simulink model "DA42_Model"  (Simulink 7.5)
settings: Solver=ode45  StartTime=0.0  StopTime=inf  RelTol=1e-3
undefined symbols (not defined in the file or in its folder): BHP_A, BHP_B, CP_norm, Pr_Alt, PropEff_norm, S
libraries: simulink_extras x4, aerolibatmos2 x2
(part 1 of 3)
settings Model: Creator=eagle  LastModifiedBy=eagle

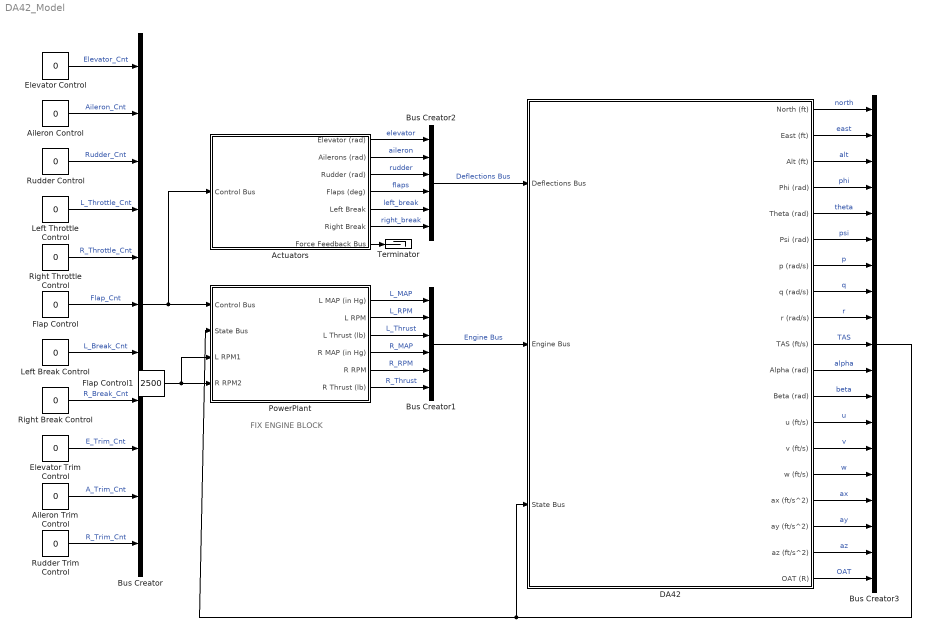
== system DA42_Model ==
  note: FIX ENGINE BLOCK
  Actuators : Subsystem
  Aileron Control : Constant  Value=0  OutDataType=sfix(16)  OutScaling=2^0
  Aileron Trim Control : Constant  Value=0  OutDataType=sfix(16)  OutScaling=2^0
  Bus Creator : BusCreator  Inputs='Elevator_Cnt','Aileron_Cnt','Rudder_Cnt','L_Throttle_Cnt','R_Throttle_Cnt','Flap_Cnt','L_Break_Cnt','R_Break_Cnt','E_Trim_Cnt','A_Trim_Cnt','R_Trim_Cnt'
  Bus Creator1 : BusCreator  Inputs='L_MAP','L_RPM','L_Thrust','R_MAP','R_RPM','R_Thrust'
  Bus Creator2 : BusCreator  Inputs='elevator','aileron','rudder','flaps','left_break','right_break'
  Bus Creator3 : BusCreator  Inputs='north','east','alt','phi','theta','psi','p','q','r','TAS','alpha','beta','u','v','w','ax','ay','az','OAT'
  DA42 : Subsystem  mask(6DoF Simulator){x0=[165               0      21.4681707               0               0               0               0     0.129383298               0               0               0           10000], Geom=[175.3 44 4.17 3935 6163.91 1029.56 5646.43 0], cg=[-7.8750 0 0.856], ac=[-7.8750 0 0.856], engR=[-3.585  5.338 0], engL=[-3.585 -5.338 0], thrustPercent=[0.966898954 0 -0.033101045], liftder=[0 0 0 -41.807 0.7530], sideder=[-0.28 -0.3940], rollder=[-0.13 -0.76 0.1180 -0.19 -0.0095], pitchder=[-0.51 0 -9.67 -0.57], yawder=[0.058 -0.11 -0.114 -0.0033 0.077]}
      mask prompts: x0 "Initial Conditions: [u v w p q r bank pitch heading N E H]"; Geom "Geometry: [S b cbar W Jx Jy Jz Jxz]"; cg "CG Location: [x y z]"; ac "AC Location: [x y z]"; engR "Right Engine Location: [x y z]"; engL "Left Engine Location: [x y z]"; thrustPercent "Thrust Percent: [x y z]"; liftder "Lift Derivatives: [CLo CLa CLadot CLq CLde]"; sideder "Side Force Derivatives: [CYb CYdr]"; rollder "Rolling Moment Derivatives: [CLb CLp CLr CLda CLdr]"; pitchder "Pitching Moment Derivatives: [Cma Cmadot Cmq Cmde]"; yawder "Yawing Moment Derivatives: [CNb CNp CNr CNda CNdr]"
      mask help:
      | 6 Degrees of Freedom simulator.
      |
      | Control Inputs = [elevator ailerons rudder throttle] rad
      mask TabNameString: Initial Conditions,Geometry,Geometry,Geometry,Engine,Engine,Engine,Derivatives,Derivatives,Derivatives,Derivatives,Derivatives
  Elevator Control : Constant  Value=0  OutDataType=sfix(16)  OutScaling=2^0
  Elevator Trim Control : Constant  Value=0  OutDataType=sfix(16)  OutScaling=2^0
  Flap Control : Constant  Value=0  OutDataType=sfix(16)  OutScaling=2^0
  Flap Control1 : Constant  Value=2500  OutDataType=sfix(16)  OutScaling=2^0
  Left Break Control : Constant  Value=0  OutDataType=sfix(16)  OutScaling=2^0
  Left Throttle Control : Constant  Value=0  OutDataType=sfix(16)  OutScaling=2^0
  PowerPlant : Subsystem  InitFcn=|
      | pitch_Angles = 15:5:40;
      | newData1 = load('-mat', 'CP_norm');
      | % Create new variables in the base workspace from those fields.
      | vars = fieldnames(newData1);
      | for i = 1:length(vars)
      |     assignin('base', vars{i}, newData1.(vars{i}));
      | end
      | clear i newData1 vars;
      | newData1 = load('-mat', 'PropEff_norm');
      | % Create new variables in the base workspace from those fields.
      | vars = fieldnames(newData1);
      | for i = 1:length(vars)
      |     assignin('base', vars{i}, newData1.(vars{i}));
      | end
      | clear i newData1 vars;
      | %% Lycoming IO-360 ENGINE PERFORMANCE
      | MAP = 12:2:28;
      | RPM = [2000; 2200; 2400; 2600; 2700];
      | %Table1:
      |     %Known: MAP and RPM.
      |     %Output: BHP-A
      |     BHP_A = [...
      |          58.0,  65.0,  68.0,  69.7,  71.5;...
      |          67.0,  75.5,  80.5,  85.0,  86.0;...
      |          79.0,  86.0,  92.5,  97.0,  99.0;...
      |          89.0,  97.0, 105.0, 110.5, 114.5;...
      |          98.0, 108.0, 116.0, 124.0, 126.0;...
      |         108.5, 118.5, 127.0, 135.5, 139.8;...
      |         118.0, 128.0, 139.0, 148.0, 152.5;...
      |         128.0, 139.0, 149.0, 160.0, 165.0;...
      |         137.5, 148.5, 161.0, 172.0, 177.5;...
      |         ];
      | %Table 2:
      |     %Known: MAP and RPM
      |     %Output: BHP-B
      |     %Comments: Equations for the lines based on linear extrapolation for
      |     %BHP-B. Has associated Excel File: "BHB_B.xlsx" to figure out the
      |     %equations for the lines
      |     for i = 1:9
      |         BHP_B(i,:) = [...
      |             ((6.818*MAP(i)) - 55.91),...
      |             ((7.167*MAP(i)) - 55.67),...
      |             ((7.857*MAP(i)) - 62.86),...
      |             ((8.333*MAP(i)) - 63.33),...
      |             ((8.5*MAP(i)) - 63),...
      |             ];
      |     end
      |     clear i;
      | %Table 3:
      |     %Known: MAP and RPM
      |     %Output: Pressure Altitude - A
      |     Pr_Alt = [...
      |         22.80, 22.70, 26.00, 25.00, 25.00;...
      |         19.20, 19.15, 19.10, 19.05, 19.00;...
      |         15.90, 15.80, 15.70, 15.60, 15.60;...
      |         12.95, 12.90, 12.80, 12.60, 12.55;...
      |         10.30, 10.25, 10.20, 10.10, 10.05;...
      |          7.85,  7.75,  7.65,  7.55,  7.50;...
      |          5.50,  5.47,  5.30,  5.25,  5.20;...
      |          3.40,  3.30,  3.25,  3.20,  3.15;...
      |          1.30,  1.25,  1.20,  1.10,  1.05;...
      |         ];
      |     Pr_Alt = Pr_Alt * 1000;
  Right Break Control : Constant  Value=0  OutDataType=sfix(16)  OutScaling=2^0
  Right Throttle Control : Constant  Value=0  OutDataType=sfix(16)  OutScaling=2^0
  Rudder Control : Constant  Value=0  OutDataType=sfix(16)  OutScaling=2^0
  Rudder Trim Control : Constant  Value=0  OutDataType=sfix(16)  OutScaling=2^0
  Terminator : Terminator
  wires:
  Aileron Control/1 -> Bus Creator/2  "Aileron_Cnt"
  Rudder Control/1 -> Bus Creator/3  "Rudder_Cnt"
  Left Throttle Control/1 -> Bus Creator/4  "L_Throttle_Cnt"
  Right Throttle Control/1 -> Bus Creator/5  "R_Throttle_Cnt"
  Flap Control/1 -> Bus Creator/6  "Flap_Cnt"
  Left Break Control/1 -> Bus Creator/7  "L_Break_Cnt"
  Right Break Control/1 -> Bus Creator/8  "R_Break_Cnt"
  Elevator Trim Control/1 -> Bus Creator/9  "E_Trim_Cnt"
  Aileron Trim Control/1 -> Bus Creator/10  "A_Trim_Cnt"
  Rudder Trim Control/1 -> Bus Creator/11  "R_Trim_Cnt"
  Elevator Control/1 -> Bus Creator/1  "Elevator_Cnt"
  PowerPlant/1(L MAP (in Hg)) -> Bus Creator1/1  "L_MAP"
  PowerPlant/2(L RPM) -> Bus Creator1/2  "L_RPM"
  PowerPlant/3(L Thrust (lb)) -> Bus Creator1/3  "L_Thrust"
  PowerPlant/4(R MAP (in Hg)) -> Bus Creator1/4  "R_MAP"
  PowerPlant/5(R RPM) -> Bus Creator1/5  "R_RPM"
  PowerPlant/6(R Thrust (lb)) -> Bus Creator1/6  "R_Thrust"
  Actuators/1(Elevator (rad)) -> Bus Creator2/1  "elevator"
  Actuators/2(Ailerons (rad)) -> Bus Creator2/2  "aileron"
  Actuators/3(Rudder (rad)) -> Bus Creator2/3  "rudder"
  Actuators/4(Flaps (deg)) -> Bus Creator2/4  "flaps"
  Actuators/5(Left Break) -> Bus Creator2/5  "left_break"
  Actuators/6(Right Break) -> Bus Creator2/6  "right_break"
  Actuators/7(Force Feedback Bus) -> Terminator/1
  Bus Creator2/1 -> DA42/1(Deflections Bus)  "Deflections Bus"
  Bus Creator1/1 -> DA42/2(Engine Bus)  "Engine Bus"
  DA42/1(North (ft)) -> Bus Creator3/1  "north"
  DA42/2(East (ft)) -> Bus Creator3/2  "east"
  DA42/3(Alt (ft)) -> Bus Creator3/3  "alt"
  DA42/4(Phi (rad)) -> Bus Creator3/4  "phi"
  DA42/5(Theta (rad)) -> Bus Creator3/5  "theta"
  DA42/6(Psi (rad)) -> Bus Creator3/6  "psi"
  DA42/7(p (rad/s)) -> Bus Creator3/7  "p"
  DA42/8(q (rad/s)) -> Bus Creator3/8  "q"
  DA42/9(r (rad/s)) -> Bus Creator3/9  "r"
  DA42/10(TAS (ft/s)) -> Bus Creator3/10  "TAS"
  DA42/11(Alpha (rad)) -> Bus Creator3/11  "alpha"
  DA42/12(Beta (rad)) -> Bus Creator3/12  "beta"
  DA42/13(u (ft/s)) -> Bus Creator3/13  "u"
  DA42/14(v (ft/s)) -> Bus Creator3/14  "v"
  DA42/15(w (ft/s)) -> Bus Creator3/15  "w"
  DA42/16(ax (ft/s^2)) -> Bus Creator3/16  "ax"
  DA42/17(ay (ft/s^2)) -> Bus Creator3/17  "ay"
  DA42/18(az (ft/s^2)) -> Bus Creator3/18  "az"
  Bus Creator3/1 -> DA42/3(State Bus), PowerPlant/2(State Bus)
  Bus Creator/1 -> PowerPlant/1(Control Bus), Actuators/1(Control Bus)
  DA42/19(OAT (R)) -> Bus Creator3/19  "OAT"
  Flap Control1/1 -> PowerPlant/4(R RPM2), PowerPlant/3(L RPM1)

== system DA42_Model/Actuators ==
  note: Orange = SR22 = Needs Updating
  Control Bus : Inport
  Aileron Control Model : Subsystem
  Aileron Trim : Subsystem
  Bus Creator1 : BusCreator  Inputs='Stick_Force','Aileron_Torque','Pedal_Force'
  Elevator Control Model : Subsystem
  Elevator Trim : Subsystem
  Flaps : Subsystem
  Left Brake : Subsystem
  Right Brake : Subsystem
  Rudder Control Model : Subsystem
  Elevator (rad) : Outport  OutDataType=fixdt(1, 16)  OutScaling=2^0
  Ailerons (rad) : Outport  Port=2  OutDataType=fixdt(1, 16)  OutScaling=2^0
  Rudder (rad) : Outport  Port=3  OutDataType=fixdt(1, 16)  OutScaling=2^0
  Flaps (deg) : Outport  Port=4  OutDataType=fixdt(1, 16)  OutScaling=2^0
  Left Break : Outport  Port=5  OutDataType=fixdt(1, 16)  OutScaling=2^0
  Right Break : Outport  Port=6  OutDataType=fixdt(1, 16)  OutScaling=2^0
  Force Feedback Bus : Outport  Port=7  OutDataType=fixdt(1, 16)  OutScaling=2^0
  wires:
  Control Bus/1 -> Elevator Control Model/1(Elevator Control), Aileron Control Model/1(Aileron Control), Right Brake/1(R_BRK_ Control), Left Brake/1(L_BRK_ Control), Flaps/1(Flap CMD), Rudder Control Model/1(Rudder Control), Aileron Trim/1(Aileron Trim CMD), Elevator Trim/1(Elevator Trim CMD)
  Flaps/1(Flap Surface) -> Rudder Control Model/4(Flap Surface), Aileron Control Model/5(Flap Surface), Elevator Control Model/5(Flap Surface), Flaps/2(Flap Surf), Flaps (deg)/1  "flaps"
  Elevator Trim/1(Elevator Trim Position) -> Elevator Trim/4(Elev Trim Position), Elevator Control Model/2(Elevator Trim Position)
  Aileron Trim/1(Aileron Trim Position) -> Aileron Trim/4(Ail Trim Position), Aileron Control Model/2(Aileron Trim Position)
  Elevator Control Model/1(Elevator Surface) -> Elevator (rad)/1  "elevator"
  Aileron Control Model/1(Aileron Torque) -> Bus Creator1/2  "Aileron_Torque"
  Rudder Control Model/1(Pedal Force) -> Bus Creator1/3  "Pedal_Force"
  Elevator Control Model/2(Stick Force) -> Bus Creator1/1  "Stick_Force"
  Bus Creator1/1 -> Force Feedback Bus/1
  Aileron Control Model/2(Aileron Surface) -> Ailerons (rad)/1  "aileron"
  Rudder Control Model/2(Rudder Surface) -> Rudder (rad)/1  "rudder"
  Right Brake/1(R_BRK_CMD) -> Right Break/1  "right_break"
  Left Brake/1(L_BRK_CMD) -> Left Break/1  "left_break"

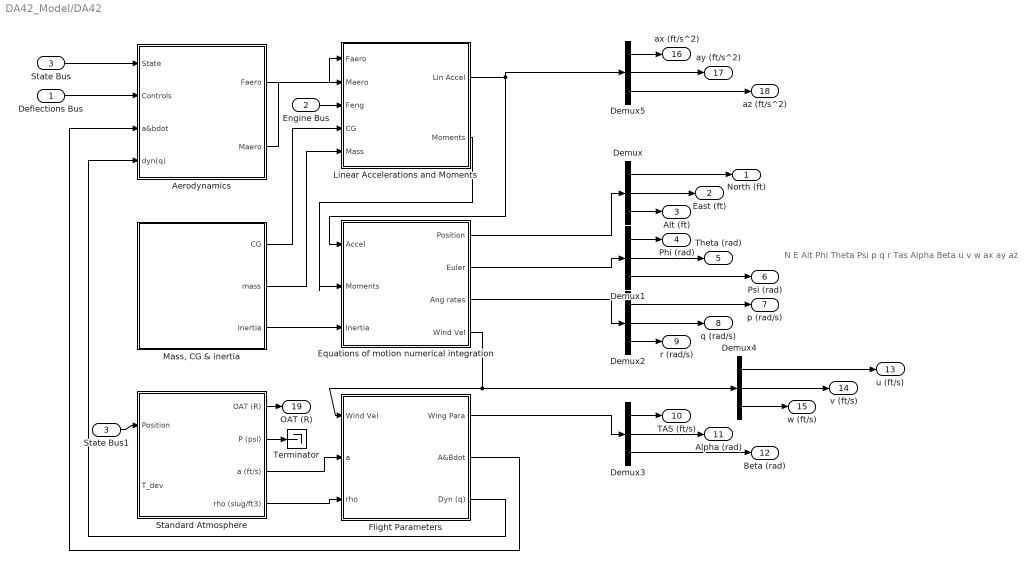
== system DA42_Model/DA42 ==
  note: N
      | E
      | Alt
      | Phi
      | Theta
      | Psi
      | p
      | q
      | r
      | Tas
      | Alpha
      | Beta
      | u
      | v
      | w
      | ax
      | ay
      | az
  Deflections Bus : Inport
  Engine Bus : Inport  Port=2
  State Bus : Inport  Port=3
  Aerodynamics : Subsystem
  Demux{,1..5} (6 alike) : Demux  Outputs=3
  "Equations of motion numerical integration " : Subsystem
  Flight Parameters : Subsystem
  Linear Accelerations and Moments : Subsystem
  "Mass, CG & inertia" : Subsystem
  Standard Atmosphere : Subsystem
  State Bus1 : InportShadow  Port=3
  Terminator : Terminator
  North (ft) : Outport
  East (ft) : Outport  Port=2
  Alt (ft) : Outport  Port=3
  Phi (rad) : Outport  Port=4
  Theta (rad) : Outport  Port=5
  Psi (rad) : Outport  Port=6
  p (rad/s) : Outport  Port=7
  q (rad/s) : Outport  Port=8
  r (rad/s) : Outport  Port=9
  TAS (ft/s) : Outport  Port=10
  Alpha (rad) : Outport  Port=11
  Beta (rad) : Outport  Port=12
  u (ft/s) : Outport  Port=13
  v (ft/s) : Outport  Port=14
  w (ft/s) : Outport  Port=15
  ax (ft/s^2) : Outport  Port=16
  ay (ft/s^2) : Outport  Port=17
  az (ft/s^2) : Outport  Port=18
  OAT (R) : Outport  Port=19
  wires:
  "Equations of motion numerical integration "/1(Position) -> Demux/1
  Flight Parameters/2(A&Bdot) -> Aerodynamics/3(a&bdot)
  Flight Parameters/3(Dyn (q)) -> Aerodynamics/4(dyn(q))
  Flight Parameters/1(Wing Para) -> Demux3/1
  "Equations of motion numerical integration "/4(Wind Vel) -> Demux4/1, Flight Parameters/1(Wind Vel)
  "Equations of motion numerical integration "/3(Ang rates) -> Demux2/1
  Linear Accelerations and Moments/1(Lin Accel) -> "Equations of motion numerical integration "/1(Accel), Demux5/1
  Deflections Bus/1 -> Aerodynamics/2(Controls)
  Aerodynamics/2(Maero) -> Linear Accelerations and Moments/2(Maero)
  Aerodynamics/1(Faero) -> Linear Accelerations and Moments/1(Faero)
  Engine Bus/1 -> Linear Accelerations and Moments/3(Feng)
  Demux/1 -> North (ft)/1
  Demux/2 -> East (ft)/1
  Demux/3 -> Alt (ft)/1
  "Equations of motion numerical integration "/2(Euler) -> Demux1/1
  Demux1/1 -> Phi (rad)/1
  Demux1/2 -> Theta (rad)/1
  Demux1/3 -> Psi (rad)/1
  Demux2/1 -> p (rad/s)/1
  Demux2/2 -> q (rad/s)/1
  Demux2/3 -> r (rad/s)/1
  Demux3/1 -> TAS (ft/s)/1
  Demux3/2 -> Alpha (rad)/1
  Demux3/3 -> Beta (rad)/1
  Demux4/1 -> u (ft/s)/1
  Demux4/2 -> v (ft/s)/1
  Demux4/3 -> w (ft/s)/1
  Demux5/1 -> ax (ft/s^2)/1
  Demux5/2 -> ay (ft/s^2)/1
  Demux5/3 -> az (ft/s^2)/1
  Linear Accelerations and Moments/2(Moments) -> "Equations of motion numerical integration "/2(Moments)
  "Mass, CG & inertia"/1(CG) -> Linear Accelerations and Moments/4(CG)
  "Mass, CG & inertia"/2(mass) -> Linear Accelerations and Moments/5(Mass)
  "Mass, CG & inertia"/3(Inertia) -> "Equations of motion numerical integration "/3(Inertia)
  Standard Atmosphere/4(rho (slug/ft3)) -> Flight Parameters/3(rho)
  Standard Atmosphere/3(a (ft/s)) -> Flight Parameters/2(a)
  State Bus/1 -> Aerodynamics/1(State)
  State Bus1/1 -> Standard Atmosphere/1(Position)
  Standard Atmosphere/1(OAT (R)) -> OAT (R)/1
  Standard Atmosphere/2(P (psi)) -> Terminator/1

== system DA42_Model/PowerPlant ==
  Control Bus : Inport
  State Bus : Inport  Port=2
  L RPM1 : Inport  Port=3
  R RPM2 : Inport  Port=4
  Bus Selector : BusSelector  OutputSignals=L_Throttle_Cnt,R_Throttle_Cnt
  Bus Selector1 : BusSelector  OutputSignals=alt,OAT,TAS
  Bus Selector2 : BusSelector  OutputSignals=alt,OAT
  Lycoming IO-1 : Subsystem  InitFcn=|
      | pitch_Angles = 15:5:40;
      | newData1 = load('-mat', 'CP_norm');
      | % Create new variables in the base workspace from those fields.
      | vars = fieldnames(newData1);
      | for i = 1:length(vars)
      |     assignin('base', vars{i}, newData1.(vars{i}));
      | end
      | clear i newData1 vars;
      | newData1 = load('-mat', 'PropEff_norm');
      | % Create new variables in the base workspace from those fields.
      | vars = fieldnames(newData1);
      | for i = 1:length(vars)
      |     assignin('base', vars{i}, newData1.(vars{i}));
      | end
      | clear i newData1 vars;
      | %% Lycoming IO-360 ENGINE PERFORMANCE
      | MAP = 12:2:28;
      | RPM = [2000; 2200; 2400; 2600; 2700];
      | %Table1:
      |     %Known: MAP and RPM.
      |     %Output: BHP-A
      |     BHP_A = [...
      |          58.0,  65.0,  68.0,  69.7,  71.5;...
      |          67.0,  75.5,  80.5,  85.0,  86.0;...
      |          79.0,  86.0,  92.5,  97.0,  99.0;...
      |          89.0,  97.0, 105.0, 110.5, 114.5;...
      |          98.0, 108.0, 116.0, 124.0, 126.0;...
      |         108.5, 118.5, 127.0, 135.5, 139.8;...
      |         118.0, 128.0, 139.0, 148.0, 152.5;...
      |         128.0, 139.0, 149.0, 160.0, 165.0;...
      |         137.5, 148.5, 161.0, 172.0, 177.5;...
      |         ];
      | %Table 2:
      |     %Known: MAP and RPM
      |     %Output: BHP-B
      |     %Comments: Equations for the lines based on linear extrapolation for
      |     %BHP-B. Has associated Excel File: "BHB_B.xlsx" to figure out the
      |     %equations for the lines
      |     for i = 1:9
      |         BHP_B(i,:) = [...
      |             ((6.818*MAP(i)) - 55.91),...
      |             ((7.167*MAP(i)) - 55.67),...
      |             ((7.857*MAP(i)) - 62.86),...
      |             ((8.333*MAP(i)) - 63.33),...
      |             ((8.5*MAP(i)) - 63),...
      |             ];
      |     end
      |     clear i;
      | %Table 3:
      |     %Known: MAP and RPM
      |     %Output: Pressure Altitude - A
      |     Pr_Alt = [...
      |         22.80, 22.70, 26.00, 25.00, 25.00;...
      |         19.20, 19.15, 19.10, 19.05, 19.00;...
      |         15.90, 15.80, 15.70, 15.60, 15.60;...
      |         12.95, 12.90, 12.80, 12.60, 12.55;...
      |         10.30, 10.25, 10.20, 10.10, 10.05;...
      |          7.85,  7.75,  7.65,  7.55,  7.50;...
      |          5.50,  5.47,  5.30,  5.25,  5.20;...
      |          3.40,  3.30,  3.25,  3.20,  3.15;...
      |          1.30,  1.25,  1.20,  1.10,  1.05;...
      |         ];
      |     Pr_Alt = Pr_Alt * 1000;
  Lycoming IO-360 : Subsystem  InitFcn=|
      | pitch_Angles = 15:5:40;
      | newData1 = load('-mat', 'CP_norm');
      | % Create new variables in the base workspace from those fields.
      | vars = fieldnames(newData1);
      | for i = 1:length(vars)
      |     assignin('base', vars{i}, newData1.(vars{i}));
      | end
      | clear i newData1 vars;
      | newData1 = load('-mat', 'PropEff_norm');
      | % Create new variables in the base workspace from those fields.
      | vars = fieldnames(newData1);
      | for i = 1:length(vars)
      |     assignin('base', vars{i}, newData1.(vars{i}));
      | end
      | clear i newData1 vars;
      | %% Lycoming IO-360 ENGINE PERFORMANCE
      | MAP = 12:2:28;
      | RPM = [2000; 2200; 2400; 2600; 2700];
      | %Table1:
      |     %Known: MAP and RPM.
      |     %Output: BHP-A
      |     BHP_A = [...
      |          58.0,  65.0,  68.0,  69.7,  71.5;...
      |          67.0,  75.5,  80.5,  85.0,  86.0;...
      |          79.0,  86.0,  92.5,  97.0,  99.0;...
      |          89.0,  97.0, 105.0, 110.5, 114.5;...
      |          98.0, 108.0, 116.0, 124.0, 126.0;...
      |         108.5, 118.5, 127.0, 135.5, 139.8;...
      |         118.0, 128.0, 139.0, 148.0, 152.5;...
      |         128.0, 139.0, 149.0, 160.0, 165.0;...
      |         137.5, 148.5, 161.0, 172.0, 177.5;...
      |         ];
      | %Table 2:
      |     %Known: MAP and RPM
      |     %Output: BHP-B
      |     %Comments: Equations for the lines based on linear extrapolation for
      |     %BHP-B. Has associated Excel File: "BHB_B.xlsx" to figure out the
      |     %equations for the lines
      |     for i = 1:9
      |         BHP_B(i,:) = [...
      |             ((6.818*MAP(i)) - 55.91),...
      |             ((7.167*MAP(i)) - 55.67),...
      |             ((7.857*MAP(i)) - 62.86),...
      |             ((8.333*MAP(i)) - 63.33),...
      |             ((8.5*MAP(i)) - 63),...
      |             ];
      |     end
      |     clear i;
      | %Table 3:
      |     %Known: MAP and RPM
      |     %Output: Pressure Altitude - A
      |     Pr_Alt = [...
      |         22.80, 22.70, 26.00, 25.00, 25.00;...
      |         19.20, 19.15, 19.10, 19.05, 19.00;...
      |         15.90, 15.80, 15.70, 15.60, 15.60;...
      |         12.95, 12.90, 12.80, 12.60, 12.55;...
      |         10.30, 10.25, 10.20, 10.10, 10.05;...
      |          7.85,  7.75,  7.65,  7.55,  7.50;...
      |          5.50,  5.47,  5.30,  5.25,  5.20;...
      |          3.40,  3.30,  3.25,  3.20,  3.15;...
      |          1.30,  1.25,  1.20,  1.10,  1.05;...
      |         ];
      |     Pr_Alt = Pr_Alt * 1000;
  State Bus1 : InportShadow  Port=2
  L MAP (in Hg) : Outport  OutDataType=fixdt(1, 16)  OutScaling=2^0
  L RPM : Outport  Port=2  OutDataType=fixdt(1, 16)  OutScaling=2^0
  L Thrust (lb) : Outport  Port=3  OutDataType=fixdt(1, 16)  OutScaling=2^0
  R MAP (in Hg) : Outport  Port=4  OutDataType=fixdt(1, 16)  OutScaling=2^0
  R RPM : Outport  Port=5  OutDataType=fixdt(1, 16)  OutScaling=2^0
  R Thrust (lb) : Outport  Port=6  OutDataType=fixdt(1, 16)  OutScaling=2^0
  wires:
  Control Bus/1 -> Bus Selector/1
  Bus Selector/1 -> Lycoming IO-360/1(MAP), L MAP (in Hg)/1  "<L_Throttle_Cnt>"
  Bus Selector/2 -> Lycoming IO-1/1(MAP), R MAP (in Hg)/1  "<R_Throttle_Cnt>"
  L RPM1/1 -> Lycoming IO-360/2(RPM), L RPM/1
  Lycoming IO-1/1(Thrust (lb)) -> R Thrust (lb)/1
  Lycoming IO-360/1(Thrust (lb)) -> L Thrust (lb)/1
  R RPM2/1 -> Lycoming IO-1/2(RPM), R RPM/1
  State Bus/1 -> Bus Selector1/1
  Bus Selector1/1 -> Lycoming IO-360/3(Pressure Alt (ft))  "<alt>"
  Bus Selector1/2 -> Lycoming IO-360/4(OAT (R))  "<OAT>"
  Bus Selector1/3 -> Lycoming IO-360/5(TAS (ft/s))  "<TAS>"
  State Bus1/1 -> Bus Selector2/1
  Bus Selector2/1 -> Lycoming IO-1/3(Pressure Alt (ft))  "<alt>"
  Bus Selector2/2 -> Lycoming IO-1/4(OAT (R))  "<OAT>"

== system DA42_Model/Actuators/Aileron Control Model ==
  Aileron Control : Inport
  Aileron Trim Position : Inport  Port=2
  Dynamic Pressure : Inport  Port=3
  AOA : Inport  Port=4
  Flap Surface : Inport  Port=5
  Aero Force : Subsystem
  Bus Selector : BusSelector  OutputSignals=Aileron_Cnt,Rudder_Cnt
  Interconnect Force : Subsystem
  Rate Limiter : RateLimiter  RisingSlewLimit=10  FallingSlewLimit=-10  SampleTimeMode=inherited
  Saturation : Saturate  UpperLimit=50  LowerLimit=-50
  Spring Force : Subsystem
  Sum Torques : Sum  Inputs=+++
  Surface Deflection : Subsystem
  deg2rad : Gain  Gain=1/57.3  ParameterDataType=fixdt(1, 16)  ParameterScaling=2^0  OutDataType=fixdt(1, 16)  OutScaling=2^0
  Aileron Torque : Outport
  Aileron Surface : Outport  Port=2
  wires:
  Rate Limiter/1 -> Aileron Torque/1
  Saturation/1 -> Rate Limiter/1
  Interconnect Force/1(Torque) -> Sum Torques/3
  Flap Surface/1 -> Aero Force/4(Flap Surface)
  Bus Selector/2 -> Interconnect Force/2(Rudder Control)  "<Rudder_Cnt>"
  Sum Torques/1 -> Saturation/1
  Aero Force/1(Aero Torque) -> Sum Torques/2
  Spring Force/1(Torque) -> Sum Torques/1
  AOA/1 -> Aero Force/3(AOA)
  Dynamic Pressure/1 -> Aero Force/2(Dynamic Pressure)
  Aileron Trim Position/1 -> Spring Force/2(Trim Position)
  Surface Deflection/1(Aileron Surface) -> Spring Force/1(Aileron Surface), Aero Force/1(Aileron Surface), deg2rad/1
  Aileron Control/1 -> Bus Selector/1
  Bus Selector/1 -> Surface Deflection/1(Aileron Control), Interconnect Force/1(Aileron Control)  "<Aileron_Cnt>"
  deg2rad/1 -> Aileron Surface/1

== system DA42_Model/Actuators/Aileron Trim ==
  note: Notes:
      | Pulling back is -1, TE UP
      | Pushing foward is +1, TE DOWN
      | Not moving it is 0
      | Adjust Integrator Saturations once calibration data has been changed
      | to the range of the flight data
  Aileron Trim CMD : Inport
  Ail Trim Reset : Inport  Port=2
  Ail Trim IC : Inport  Port=3
  Ail Trim Position : Inport  Port=4
  Matching Flag : Inport  Port=5
  Bus Selector : BusSelector  OutputSignals=A_Trim_Cnt
  Integrator : Integrator  ExternalReset=either  InitialConditionSource=external  LimitOutput=on  UpperSaturationLimit=4.33  LowerSaturationLimit=3.35
  Switch General/Matching : Switch  Criteria=u2 > Threshold
  "T.E. Down limit, Calibration" : Constant  Value=3.35
  "T.E. Down limit, Flight" : Constant  Value=0.45
  "T.E. UP limit, Calibration" : Constant  Value=4.33
  "T.E. UP limit, Flight" : Constant  Value=-.53
  elev motor lag1 : Gain  Gain=.0935
  Aileron Trim Position : Outport
  wires:
  Switch General/Matching/1 -> Aileron Trim Position/1
  Ail Trim Position/1 -> Switch General/Matching/1
  Integrator/1 -> Switch General/Matching/3
  Matching Flag/1 -> Switch General/Matching/2
  elev motor lag1/1 -> Integrator/1
  Ail Trim Reset/1 -> Integrator/2
  Ail Trim IC/1 -> Integrator/3
  Aileron Trim CMD/1 -> Bus Selector/1
  Bus Selector/1 -> elev motor lag1/1  "<A_Trim_Cnt>"

== system DA42_Model/Actuators/Elevator Control Model ==
  Elevator Control : Inport
  Elevator Trim Position : Inport  Port=2
  Dynamic Pressure : Inport  Port=3
  AOA : Inport  Port=4
  Flap Surface : Inport  Port=5
  Aero Model : Subsystem
  Bus Selector : BusSelector  OutputSignals=Elevator_Cnt
  Gain : Gain  Gain=180/pi
  Rate Limiter : RateLimiter  RisingSlewLimit=20  FallingSlewLimit=-20  SampleTimeMode=inherited
  Saturation : Saturate  UpperLimit=60  LowerLimit=-60
  Spring Force : Subsystem
  Sum Forces : Sum
  Surface Defection : Subsystem
  deg2rad : Gain  Gain=1/57.3  ParameterDataType=fixdt(1, 16)  ParameterScaling=2^0  OutDataType=fixdt(1, 16)  OutScaling=2^0
  Elevator Surface : Outport
  Stick Force : Outport  Port=2
  wires:
  Gain/1 -> Aero Model/3(AOA)
  AOA/1 -> Gain/1
  Surface Defection/2(Elevator Surface) -> Spring Force/1(Elevator Surface), Aero Model/1(Elevator Surface), deg2rad/1
  Flap Surface/1 -> Aero Model/4(Flap Surface)
  Aero Model/1(Aero Force) -> Sum Forces/2
  Spring Force/1(Spring Force) -> Sum Forces/1
  Dynamic Pressure/1 -> Aero Model/2(Dynamic Pressure)
  Elevator Trim Position/1 -> Surface Defection/2(Elevator Trim Position), Spring Force/2(Trim Position)
  Sum Forces/1 -> Saturation/1
  Saturation/1 -> Rate Limiter/1
  Rate Limiter/1 -> Stick Force/1
  Elevator Control/1 -> Bus Selector/1
  Bus Selector/1 -> Surface Defection/1(Elevator Control)  "<Elevator_Cnt>"
  deg2rad/1 -> Elevator Surface/1

== system DA42_Model/Actuators/Elevator Trim ==
  note: Notes:
      | Pulling back is +1, TE UP
      | Pushing foward is -1, TE DOWN
      | Not moving it is 0
      | Adjust Integrator Saturations once calibration data has been changed
      | to the range of the flight data
  Elevator Trim CMD : Inport
  Elev Trim Reset : Inport  Port=2
  Elevator Trim IC : Inport  Port=3
  Elev Trim Position : Inport  Port=4
  Matching Flag : Inport  Port=5
  Bus Selector : BusSelector  OutputSignals=E_Trim_Cnt
  Gain : Gain  Gain=0.54
  Integrator : Integrator  ExternalReset=either  InitialConditionSource=external  LimitOutput=on  UpperSaturationLimit=4.33  LowerSaturationLimit=3.378
  Switch General/Matching : Switch  Criteria=u2 > Threshold
  Switch General/Matching1 : Switch  Threshold=3.55
  "T.E. Down limit, Calibration" : Constant  Value=3.378
  "T.E. Down limit, Flight" : Constant  Value=0.45
  "T.E. UP limit, Calibration" : Constant  Value=4.33
  "T.E. UP limit, Flight" : Constant  Value=-.53
  elev motor lag1 : Gain  Gain=.0935
  Elevator Trim Position : Outport
  wires:
  Elev Trim Position/1 -> Switch General/Matching/1
  Matching Flag/1 -> Switch General/Matching/2
  Elev Trim Reset/1 -> Integrator/2
  Elevator Trim IC/1 -> Integrator/3
  Elevator Trim CMD/1 -> Bus Selector/1
  Switch General/Matching/1 -> Elevator Trim Position/1
  Integrator/1 -> Switch General/Matching1/2, Switch General/Matching/3
  elev motor lag1/1 -> Switch General/Matching1/1, Gain/1
  Switch General/Matching1/1 -> Integrator/1
  Gain/1 -> Switch General/Matching1/3
  Bus Selector/1 -> elev motor lag1/1  "<E_Trim_Cnt>"

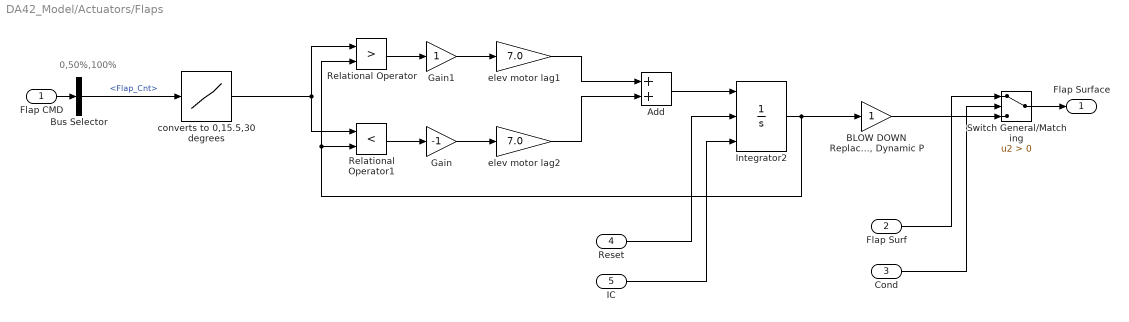
== system DA42_Model/Actuators/Flaps ==
  note: 0,50%,100%
  Flap CMD : Inport
  Flap Surf : Inport  Port=2
  Cond : Inport  Port=3
  Reset : Inport  Port=4
  IC : Inport  Port=5
  Add : Sum
  "BLOW DOWN Replace BY a LUT Function of AOA, Dynamic P" : Gain
  Bus Selector : BusSelector  OutputSignals=Flap_Cnt
  Gain : Gain  Gain=-1
  Gain1 : Gain
  Integrator2 : Integrator  ExternalReset=either  InitialConditionSource=external
  Relational Operator : RelationalOperator  Operator=>  LogicOutDataTypeMode=Specify via dialog  LogicDataType=float('double')  OutDataTypeStr=float('double')
  Relational Operator1 : RelationalOperator  Operator=<  LogicOutDataTypeMode=Specify via dialog  LogicDataType=float('double')  OutDataTypeStr=float('double')
  Switch General/Matching : Switch  Criteria=u2 > Threshold
  converts to 0,15.5,30 degrees : Lookup  InputValues=[0 50 100]  Table=[0 15.5 30]  LookUpMeth=Use Input Nearest
  elev motor lag1 : Gain  Gain=7.0
  elev motor lag2 : Gain  Gain=7.0
  Flap Surface : Outport
  wires:
  Reset/1 -> Integrator2/2
  IC/1 -> Integrator2/3
  converts to 0,15.5,30 degrees/1 -> Relational Operator1/1, Relational Operator/1
  Flap CMD/1 -> Bus Selector/1
  Integrator2/1 -> Relational Operator1/2, Relational Operator/2, "BLOW DOWN Replace BY a LUT Function of AOA, Dynamic P"/1
  Relational Operator/1 -> Gain1/1
  Relational Operator1/1 -> Gain/1
  Gain/1 -> elev motor lag2/1
  Gain1/1 -> elev motor lag1/1
  Add/1 -> Integrator2/1
  elev motor lag1/1 -> Add/1
  elev motor lag2/1 -> Add/2
  "BLOW DOWN Replace BY a LUT Function of AOA, Dynamic P"/1 -> Switch General/Matching/3
  Switch General/Matching/1 -> Flap Surface/1
  Flap Surf/1 -> Switch General/Matching/1
  Cond/1 -> Switch General/Matching/2
  Bus Selector/1 -> converts to 0,15.5,30 degrees/1  "<Flap_Cnt>"

== system DA42_Model/Actuators/Left Brake ==
  L_BRK_ Control : Inport
  Bus Selector : BusSelector  OutputSignals=L_Break_Cnt
  L_BRK_CMD : Outport
  wires:
  L_BRK_ Control/1 -> Bus Selector/1
  Bus Selector/1 -> L_BRK_CMD/1  "<L_Break_Cnt>"

== system DA42_Model/Actuators/Right Brake ==
  R_BRK_ Control : Inport
  Bus Selector : BusSelector  OutputSignals=R_Break_Cnt
  R_BRK_CMD : Outport
  wires:
  R_BRK_ Control/1 -> Bus Selector/1
  Bus Selector/1 -> R_BRK_CMD/1  "<R_Break_Cnt>"

== system DA42_Model/Actuators/Rudder Control Model ==
  Rudder Control : Inport
  Dynamic Pressure : Inport  Port=2
  Beta : Inport  Port=3
  Flap Surface : Inport  Port=4
  Aero Force : Subsystem
  Bus Selector : BusSelector  OutputSignals=Rudder_Cnt,Aileron_Cnt
  Interconnect Force : Subsystem
  Rate Limiter : RateLimiter  RisingSlewLimit=40  FallingSlewLimit=-40  SampleTimeMode=inherited
  Saturation : Saturate  UpperLimit=150  LowerLimit=-150
  Spring Force : Subsystem
  Sum Forces : Sum  Inputs=+++
  Surface Deflection : Subsystem
  deg2rad : Gain  Gain=1/57.3  ParameterDataType=fixdt(1, 16)  ParameterScaling=2^0  OutDataType=fixdt(1, 16)  OutScaling=2^0
  Pedal Force : Outport
  Rudder Surface : Outport  Port=2
  wires:
  Rate Limiter/1 -> Pedal Force/1
  Saturation/1 -> Rate Limiter/1
  Interconnect Force/1(Bungee Force) -> Sum Forces/3
  Aero Force/1(Aero Force) -> Sum Forces/2
  Flap Surface/1 -> Aero Force/4(Flap Surface)
  Spring Force/1(Pedal Force) -> Sum Forces/1
  Dynamic Pressure/1 -> Aero Force/2(Dynamic Pressure)
  Surface Deflection/1(Rudder Surface) -> Spring Force/1(Rudder Surface), Aero Force/1(Rudder Surface), deg2rad/1
  Sum Forces/1 -> Saturation/1
  Beta/1 -> Aero Force/3(Beta)
  Rudder Control/1 -> Bus Selector/1
  Bus Selector/1 -> Surface Deflection/1(Rudder Control), Interconnect Force/1(Rudder Control)  "<Rudder_Cnt>"
  Bus Selector/2 -> Interconnect Force/2(Aileron Control)  "<Aileron_Cnt>"
  deg2rad/1 -> Rudder Surface/1

== system DA42_Model/DA42/Aerodynamics ==
  State : Inport
  Controls : Inport  Port=2
  a&bdot : Inport  Port=3
  dyn(q) : Inport  Port=4
  Aero Forces and Moments : Subsystem
  CD : Subsystem
  CL : Subsystem
  CM : Subsystem
  CN : Subsystem
  CY : Subsystem
  Controls1 : InportShadow  Port=2
  Croll : Subsystem
  State1 : InportShadow  Port=1
  a&bdot1 : InportShadow  Port=3
  Faero : Outport
  Maero : Outport  Port=2
  wires:
  Aero Forces and Moments/2(Maero) -> Maero/1
  Aero Forces and Moments/1(Faero) -> Faero/1
  dyn(q)/1 -> Aero Forces and Moments/1(dyn(q))
  CM/1(CM) -> Aero Forces and Moments/7(CM)
  CY/1(CY) -> Aero Forces and Moments/3(CY)
  Croll/1(Croll) -> Aero Forces and Moments/6(Croll)
  CN/1(CN) -> Aero Forces and Moments/8(CN)
  CD/1(CD) -> Aero Forces and Moments/2(CD)
  Controls/1 -> CM/1(Controls), CL/1(Controls)
  State/1 -> CM/3(State), CL/3(State), CD/1(State)
  CL/1(CL) -> Aero Forces and Moments/4(CL)
  a&bdot/1 -> CM/2(a&bdot)
  a&bdot1/1 -> CL/2(a&bdot)
  Controls1/1 -> CY/2(Controls), Croll/1(Controls), CN/1(Controls)
  State1/1 -> CY/1(State), Croll/2(State), CN/2(State), Aero Forces and Moments/5(State)

== system DA42_Model/DA42/Equations of motion numerical integration  ==
  Accel : Inport
  Moments : Inport  Port=2
  Inertia : Inport  Port=3
  Flat Earth Navigation : Subsystem
  Force Equations : Subsystem
  Gravity Model : Subsystem
  Inert-body : Subsystem
  Kinematic Equiations : Subsystem
  Moment Equations : Subsystem
  Terminator : Terminator
  Terminator1 : Terminator
  Position : Outport
  Euler : Outport  Port=2
  Ang rates : Outport  Port=3
  Wind Vel : Outport  Port=4
  wires:
  Inert-body/1(NEDtoBC) -> Force Equations/4(NEDtoABC)
  Flat Earth Navigation/1(Position) -> Position/1
  Moments/1 -> Moment Equations/2(Moments)
  Gravity Model/1(Gravity) -> Force Equations/2(Gravity)
  Inertia/1 -> Moment Equations/1(Inertia)
  Accel/1 -> Force Equations/1(Accel)
  Force Equations/1(Lin Vel) -> Flat Earth Navigation/2(Velocity), Wind Vel/1
  Kinematic Equiations/1(Euler angles) -> Euler/1, Inert-body/1(Euler), Flat Earth Navigation/1(Euler Angles)
  Moment Equations/1(Ang Rates) -> Ang rates/1, Force Equations/3(Rates), Kinematic Equiations/1(Rates)
  Moment Equations/2(Ang Accel) -> Terminator/1
  Kinematic Equiations/2(Euler Rates) -> Terminator1/1

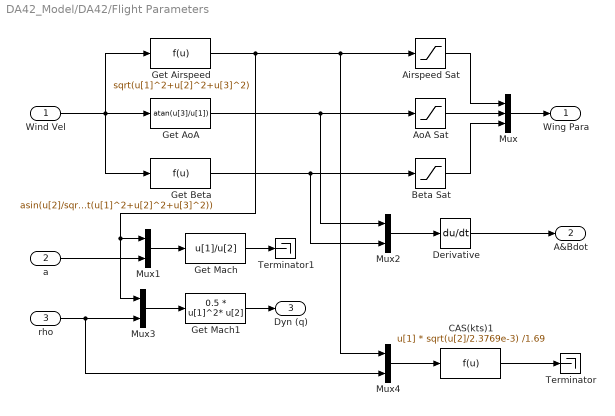
== system DA42_Model/DA42/Flight Parameters ==
  Wind Vel : Inport
  a : Inport  Port=2
  rho : Inport  Port=3
  Airspeed Sat : Saturate  UpperLimit=1100  LowerLimit=0
  AoA Sat : Saturate  UpperLimit=0.3  LowerLimit=-0.2
  Beta Sat : Saturate  UpperLimit=0.4  LowerLimit=-0.4
  CAS(kts)1 : Fcn  Expr=u[1] * sqrt(u[2]/2.3769e-3) /1.69
  Derivative : Derivative
  Get Airspeed : Fcn  Expr=sqrt(u[1]^2+u[2]^2+u[3]^2)
  Get AoA : Fcn  Expr=atan(u[3]/u[1])
  Get Beta : Fcn  Expr=asin(u[2]/sqrt(u[1]^2+u[2]^2+u[3]^2))
  Get Mach : Fcn  Expr=u[1]/u[2]
  Get Mach1 : Fcn  Expr=0.5 * u[1]^2* u[2]
  Mux : Mux  Inputs=3
  Mux{1..4} (4 alike) : Mux  Inputs=2
  Terminator : Terminator
  Terminator1 : Terminator
  Wing Para : Outport
  A&Bdot : Outport  Port=2
  Dyn (q) : Outport  Port=3
  wires:
  Mux4/1 -> CAS(kts)1/1
  Get Mach1/1 -> Dyn (q)/1
  Mux3/1 -> Get Mach1/1
  rho/1 -> Mux4/2, Mux3/2
  Get Mach/1 -> Terminator1/1
  Derivative/1 -> A&Bdot/1
  Mux2/1 -> Derivative/1
  a/1 -> Mux1/2
  Mux1/1 -> Get Mach/1
  Mux/1 -> Wing Para/1
  Beta Sat/1 -> Mux/3
  Airspeed Sat/1 -> Mux/1
  AoA Sat/1 -> Mux/2
  Get Beta/1 -> Mux2/2, Beta Sat/1
  Get AoA/1 -> Mux2/1, AoA Sat/1
  Get Airspeed/1 -> Airspeed Sat/1, Mux4/1, Mux3/1, Mux1/1
  Wind Vel/1 -> Get Beta/1, Get Airspeed/1, Get AoA/1
  CAS(kts)1/1 -> Terminator/1

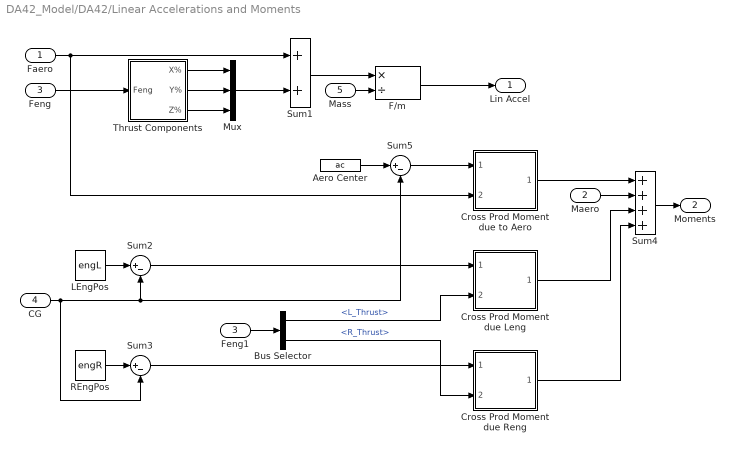
== system DA42_Model/DA42/Linear Accelerations and Moments ==
  Faero : Inport
  Maero : Inport  Port=2
  Feng : Inport  Port=3
  CG : Inport  Port=4
  Mass : Inport  Port=5
  Aero Center : Constant  Value=ac
  Bus Selector : BusSelector  OutputSignals=L_Thrust,R_Thrust
  Cross Prod Moment due Leng : Subsystem
  Cross Prod Moment due Reng : Subsystem
  Cross Prod Moment due to Aero : Subsystem
  F/m : Product  Inputs=*/  SaturateOnIntegerOverflow=on  OutDataTypeStr=Inherit: Same as first input
  Feng1 : InportShadow  Port=3
  LEngPos : Constant  Value=engL
  Mux : Mux  Inputs=3
  REngPos : Constant  Value=engR
  Sum1 : Sum  SaturateOnIntegerOverflow=on
  Sum2 : Sum  Inputs=|+-  SaturateOnIntegerOverflow=on
  Sum3 : Sum  Inputs=|+-  SaturateOnIntegerOverflow=on
  Sum4 : Sum  Inputs=++++  SaturateOnIntegerOverflow=on
  Sum5 : Sum  Inputs=|+-  SaturateOnIntegerOverflow=on
  Thrust Components : Subsystem
  Lin Accel : Outport
  Moments : Outport  Port=2
  wires:
  Cross Prod Moment due Reng/1(X Prod) -> Sum4/4
  Sum3/1 -> Cross Prod Moment due Reng/1(Vec 1)
  REngPos/1 -> Sum3/1
  LEngPos/1 -> Sum2/1
  Cross Prod Moment due Leng/1(X Prod) -> Sum4/3
  Sum2/1 -> Cross Prod Moment due Leng/1(Vec 1)
  Cross Prod Moment due to Aero/1(X Prod) -> Sum4/1
  Sum4/1 -> Moments/1
  Maero/1 -> Sum4/2
  Sum5/1 -> Cross Prod Moment due to Aero/1(Vec 1)
  Aero Center/1 -> Sum5/1
  CG/1 -> Sum3/2, Sum5/2, Sum2/2
  F/m/1 -> Lin Accel/1
  Mass/1 -> F/m/2
  Sum1/1 -> F/m/1
  Mux/1 -> Sum1/2
  Faero/1 -> Sum1/1, Cross Prod Moment due to Aero/2(Vec 2)
  Feng/1 -> Thrust Components/1(Feng)
  Thrust Components/1(X%) -> Mux/1
  Thrust Components/2(Y%) -> Mux/2
  Thrust Components/3(Z%) -> Mux/3
  Feng1/1 -> Bus Selector/1
  Bus Selector/1 -> Cross Prod Moment due Leng/2(Vec 2)  "<L_Thrust>"
  Bus Selector/2 -> Cross Prod Moment due Reng/2(Vec 2)  "<R_Thrust>"

== system DA42_Model/DA42/Mass, CG & inertia ==
  Mux1 : Mux
  cg : Constant  Value=cg
  jx : Constant  Value=Geom(5)
  jxz : Constant  Value=Geom(8)
  jy : Constant  Value=Geom(6)
  jz : Constant  Value=Geom(7)
  mass2 : Constant  Value=Geom(4)/32.2
  CG : Outport
  mass : Outport  Port=2
  Inertia : Outport  Port=3
  wires:
  mass2/1 -> mass/1
  Mux1/1 -> Inertia/1
  jxz/1 -> Mux1/4
  jz/1 -> Mux1/3
  jx/1 -> Mux1/1
  jy/1 -> Mux1/2
  cg/1 -> CG/1

== system DA42_Model/DA42/Standard Atmosphere ==
  note: From Aerospace Blockset
  Position : Inport  OutDataType=sfix(16)  OutScaling=2^0
  T_dev : Inport  Port=2  OutDataType=sfix(16)  OutScaling=2^0
  Atmosphere Model : Subsystem  mask(International Standard Atmosphere Model){custom=off, g=9.80665, gamma=1.4, R=287.0531, L=0.0065, h_trop=11000, h_strat=20000, rho0=1.225, P0=101325, T0=288.15}
      mask prompts: custom "Change atmospheric parameters"; g "Acceleration due to gravity (m/s^2):"; gamma "Ratio of specific heats:"; R "Characteristic gas constant (J/Kg/K):"; L "Lapse rate (K/m):"; h_trop "Height of troposphere (m):"; h_strat "Height of tropopause (m):"; rho0 "Air density at mean sea level (Kg/m^3):"; P0 "Ambient pressure at mean sea level (N/m^2):"; T0 "Ambient temperature at mean sea level (K):"
      mask help:
      | Compute International Standard Atmosphere (ISA) model for altitudes between 0 Km and 20 Km using a lapse rate method.
      |
      | Select change atmospheric parameters to create custom atmosphere.
      mask init:
      | ports = aeroicon('aeroblkisa','icon');
      | [x y miny txt] = aeroimage('atmosphere');
      mask Help: eval('asbhelp(''isa_atmosphere_model'')');
      mask CallbackString: aeroicon('aeroblkisa')|||||||||
      mask Display:
      | port_label('input',1,'h (m)','texmode','on');
      | port_label('output',1,'T (K)','texmode','on');
      | port_label('output',2,'a (m/s)','texmode','on');
      | port_label('output',3,'P (Pa)','texmode','on');
      | port_label('output',4,'\rho (kg/m^3)','texmode','on');
      | plot(x,y)
      | text(0.5,miny-.07,txt,'HorizontalAlignment','center');
  Bus Selector : BusSelector  OutputSignals=alt
  Kelvin 2 Rankine : Gain  Gain=1.8  ParameterDataType=sfix(16)  ParameterScaling=2^0  OutDataType=sfix(16)  OutScaling=2^0
  Pa 2 PSI : Gain  Gain=0.0001450377  ParameterDataType=sfix(16)  ParameterScaling=2^0  OutDataType=sfix(16)  OutScaling=2^0
  ft 2 m : Gain  Gain=0.3048  ParameterDataType=sfix(16)  ParameterScaling=2^0  OutDataType=sfix(16)  OutScaling=2^0
  kg/m3 2 slug/ft3 : Gain  Gain=0.00194032  ParameterDataType=sfix(16)  ParameterScaling=2^0  OutDataType=sfix(16)  OutScaling=2^0
  m/s 2 ft/s : Gain  Gain=3.280839895  ParameterDataType=sfix(16)  ParameterScaling=2^0  OutDataType=sfix(16)  OutScaling=2^0
  OAT (R) : Outport  OutDataType=sfix(16)  OutScaling=2^0
  P (psi) : Outport  Port=2  OutDataType=sfix(16)  OutScaling=2^0
  a (ft/s) : Outport  Port=3  OutDataType=sfix(16)  OutScaling=2^0
  rho (slug/ft3) : Outport  Port=4  OutDataType=sfix(16)  OutScaling=2^0
  wires:
  Position/1 -> Bus Selector/1
  Atmosphere Model/1(Temperature) -> Kelvin 2 Rankine/1
  Atmosphere Model/2(Speed of Sound) -> m/s 2 ft/s/1
  Atmosphere Model/4(Air Density) -> kg/m3 2 slug/ft3/1
  Atmosphere Model/3(Air Pressure) -> Pa 2 PSI/1
  ft 2 m/1 -> Atmosphere Model/1(Height)
  kg/m3 2 slug/ft3/1 -> rho (slug/ft3)/1
  Pa 2 PSI/1 -> P (psi)/1
  Kelvin 2 Rankine/1 -> OAT (R)/1
  T_dev/1 -> Atmosphere Model/2(Height1)
  m/s 2 ft/s/1 -> a (ft/s)/1
  Bus Selector/1 -> ft 2 m/1  "<alt>"

== system DA42_Model/PowerPlant/Lycoming IO-1 ==
  MAP : Inport
  RPM : Inport  Port=2
  Pressure Alt (ft) : Inport  Port=3
  OAT (R) : Inport  Port=4
  Prop Efficiency  with Cp input : Subsystem
  Rankine To Celsius : Fcn  Expr=5*(u(1)-491.67)/9
  Subsystem : Subsystem
  Thrust : Subsystem
  Thrust (lb) : Outport
  tag scope: Cp_right=global
  wires:
  Thrust/1("Thrust ") -> Thrust (lb)/1
  Rankine To Celsius/1 -> Subsystem/4(Inlet temp C)
  OAT (R)/1 -> Rankine To Celsius/1
  Pressure Alt (ft)/1 -> Subsystem/3(Pressure alt)
  [TAS] -> Prop Efficiency  with Cp input/1(TAS)
  [RPS_right] -> Prop Efficiency  with Cp input/2(RPS)
  [Prop_D_right] -> Prop Efficiency  with Cp input/3(Prop D)
  [BHP_E_right] -> Thrust/2(BHP E)
  [n_right] -> Thrust/3(n)
  [TAS] -> Thrust/1(TAS)
  Prop Efficiency  with Cp input/1(n) -> [n_right]
  Subsystem/1(Cp) -> [Cp_right]
  MAP/1 -> Subsystem/1(Map)
  RPM/1 -> Subsystem/2(RPM1)

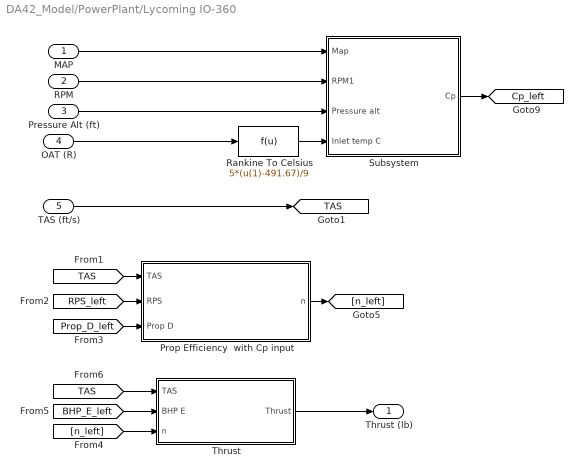
== system DA42_Model/PowerPlant/Lycoming IO-360 ==
  MAP : Inport
  RPM : Inport  Port=2
  Pressure Alt (ft) : Inport  Port=3
  OAT (R) : Inport  Port=4
  TAS (ft/s) : Inport  Port=5
  Prop Efficiency  with Cp input : Subsystem
  Rankine To Celsius : Fcn  Expr=5*(u(1)-491.67)/9
  Subsystem : Subsystem
  Thrust : Subsystem
  Thrust (lb) : Outport
  tag scope: Cp_left=global, TAS=global
  wires:
  RPM/1 -> Subsystem/2(RPM1)
  MAP/1 -> Subsystem/1(Map)
  Subsystem/1(Cp) -> [Cp_left]
  Prop Efficiency  with Cp input/1(n) -> [n_left]
  [TAS] -> Thrust/1(TAS)
  [n_left] -> Thrust/3(n)
  [BHP_E_left] -> Thrust/2(BHP E)
  [Prop_D_left] -> Prop Efficiency  with Cp input/3(Prop D)
  [RPS_left] -> Prop Efficiency  with Cp input/2(RPS)
  [TAS] -> Prop Efficiency  with Cp input/1(TAS)
  Pressure Alt (ft)/1 -> Subsystem/3(Pressure alt)
  OAT (R)/1 -> Rankine To Celsius/1
  TAS (ft/s)/1 -> [TAS]
  Rankine To Celsius/1 -> Subsystem/4(Inlet temp C)
  Thrust/1("Thrust ") -> Thrust (lb)/1

== system DA42_Model/Actuators/Aileron Control Model/Aero Force ==
  Aileron Surface : Inport
  Dynamic Pressure : Inport  Port=2
  AOA : Inport  Port=3
  Flap Surface : Inport  Port=4
  Ch : Sum  Inputs=+++
  Ch_AOA1 : Lookup2D  RowIndex=[-1.923457087514 -1.12132420883056 -0.504298917535596 -0.028307978536628 0.60634660679533 1.85802648342225 3.07444777197517 4.23798117841709 5.94797367594456]  ColumnIndex=[0 15 30]  Table=[0.00103021978021978 0.000891941391941392 0.000782967032967033;0.000552197802197802 0.000423076923076923 0.000337912087912088;0.000255494505494506 0.00015934065934066 7.41758241758241e-005;4.12087912087912e-005 -7.50915750915748e-005 -0.00014010989010989;-0.000206043956043956 -0.000288461538461539 -0.000370879120879121;-0.00070054945054945 -0.000782967032967033 -0.000865384615384616;-0.00111263736263736 -0.00121153846153846 -0.00129395604395604;-0.00159065934065934 -0.00167216117216117 -0.00175549450549451;-0.00241483516483517 -0.00251373626373626 -0.00257967032967033]
  Ch_dela1 : Lookup2D  RowIndex=[-3.03844044511145 -2.43601863211326 -1.74753656011533 -1.35195827129961 -1.17123915045212 -1.02731421914972 -0.910325967208379 -0.71234584853842 -0.424374766836659 0.295552937417741 1.01998018982373]  ColumnIndex=[0 15 30]  Table=[0.00239010989010989 0.00896703296703297 0.0076588486140725;0.00252197802197802 0.00826373626373626 0.00709594882729211;0.00242307692307692 0.00668131868131868 0.00591897654584222;0.00192857142857143 0.00523076923076923 0.0047032967032967;0.00146703296703297 0.00439005601352365 0.00328358208955224;0.00123626373626374 0.00396896003686582 0.00213219616204691;0.00110439560439561 0.00366483516483516 0.00169722814498934;0.000939560439560441 0.00315979782652379 0.0015;0.00080769230769231 0.00252564102564103 0.00126923076923077;0.00047802197802198 0.00130952380952381 0.000801705756929639;0.000214285714285712 0.000265567765567767 0.000417910447761195]
  Constant : Constant  Value=0
  Gain : Gain  Gain=-1
  Gain1 : Gain  Gain=180/pi
  Hinge Moment : Product  RndMeth=Zero
  Product : Product  RndMeth=Zero
  Wing Area : Constant  Value=S
  Aero Torque : Outport
  wires:
  Gain1/1 -> Ch_AOA1/1
  Constant/1 -> Ch/3
  Hinge Moment/1 -> Aero Torque/1
  Gain/1 -> Ch_dela1/1
  Aileron Surface/1 -> Gain/1
  Ch_dela1/1 -> Ch/1
  Ch_AOA1/1 -> Ch/2
  AOA/1 -> Gain1/1
  Flap Surface/1 -> Ch_AOA1/2, Ch_dela1/2
  Dynamic Pressure/1 -> Product/1
  Wing Area/1 -> Product/2
  Ch/1 -> Hinge Moment/2
  Product/1 -> Hinge Moment/1

== system DA42_Model/Actuators/Aileron Control Model/Interconnect Force ==
  Aileron Control : Inport
  Rudder Control : Inport  Port=2
  Aileron Cable Displacement (in) : Lookup  InputValues=|  Table=|
      InputValues=|
      | [-33.4770	
      | -27.7272	
      | -22.1070	
      | -14.5237	
      | -7.2592	
      | -0.0745	
      | 7.0405	
      | 13.6672	
      | 20.0049	
      | 26.1632	
      | 32.4012	
      | 38.8884]
      Table=|
      | [1.082677165	
      | 0.885826772	
      | 0.688976378	
      | 0.492125984	
      | 0.295275591	
      | 0.098425197	
      | -0.098425197	
      | -0.295275591	
      | -0.492125984	
      | -0.688976378	
      | -0.885826772	
      | -1.082677165]
  Bungee Torque (in-lbs) : Lookup  InputValues=[-0.899572649677258 -0.524405934143209 -0.211691388223675 -0.0927717721697674 -0.0321577688537226 0 0.0172403302966602 0.0577533517652129 0.194418255105995 0.460555172138045 1.01494242922126]  Table=[19.9725274725275 20.1373626373626 19.6428571428571 19.1483516483516 16.7032967032967 0 -11.7032967032967 -15.3846153846154 -18.4615384615385 -19.3406593406594 -19.9175824175824]
  DeadBand : DeadZone  LowerValue=-1  UpperValue=1  SaturateOnIntegerOverflow=on
  Interconect Delta (in) : Sum  Inputs=-+
  Rudder Cable Displacement (in) : Lookup  InputValues=|  Table=|
      InputValues=|
      | [-49	
      | -42.5	
      | -32	
      | -23.5	
      | -11.25	
      | 0	
      | 8	
      | 14.5	
      | 20.5	
      | 26	
      | 31.25	
      | 33.5]
      Table=|
      | [-0.86614	
      | -0.7874	
      | -0.59055	
      | -0.3937	
      | -0.19685	
      | 0	
      | 0.19685	
      | 0.3937	
      | 0.59055	
      | 0.7874	
      | 0.98425	
      | 1.082675]
  Torque : Outport
  wires:
  Bungee Torque (in-lbs)/1 -> Torque/1
  Interconect Delta (in)/1 -> DeadBand/1
  DeadBand/1 -> Bungee Torque (in-lbs)/1
  Rudder Cable Displacement (in)/1 -> Interconect Delta (in)/2
  Rudder Control/1 -> Rudder Cable Displacement (in)/1
  Aileron Cable Displacement (in)/1 -> Interconect Delta (in)/1
  Aileron Control/1 -> Aileron Cable Displacement (in)/1

== system DA42_Model/Actuators/Aileron Control Model/Spring Force ==
  Aileron Surface : Inport
  Trim Position : Inport  Port=2
  Aileron Trim Position (in) : Lookup  InputValues=[-2.45 0 6.97]  Table=[0.19 0 -0.47]
  Spring Delta (in) : Sum  Inputs=-+
  Torque (in-lbs) : Lookup  InputValues=|  Table=|
      InputValues=|
      | [-0.9318	
      | -0.9298	
      | -0.9198	
      | -0.8991	
      | -0.8726	
      | -0.8464	
      | -0.8213	
      | -0.7958	
      | -0.7699	
      | -0.7446	
      | -0.7194	
      | -0.692	
      | -0.6626	
      | -0.6334	
      | -0.6054	
      | -0.5773	
      | -0.5478	
      | -0.5178	
      | -0.4878	
      | -0.4586	
      | -0.4311	
      | -0.4036	
      | -0.3742	
      | -0.3432	
      | -0.3094	
      | -0.2717	
      | -0.232	
      | -0.192	
      | -0.1505	
      | -0.1081	
      | -0.0692	
      | -0.0391	
      | -0.0205	
      | -0.0093	
      | 0.0007	
      | 0.0102	
      | 0.0236	
      | 0.0437	
      | 0.0642	
      | 0.0825	
      | 0.1029	
      | 0.1269	
      | 0.1528	
      | 0.1767	
      | 0.1965	
      | 0.2136	
      | 0.2295	
      | 0.2467	
      | 0.2651	
      | 0.2828	
      | 0.301	
      | 0.3208	
      | 0.3408	
      | 0.3587	
      | 0.3762	
      | 0.3958	
      | 0.4171	
      | 0.4394	
      | 0.4625	
      | 0.4872	
      | 0.5152	
      | 0.5457	
      | 0.577	
      | 0.6082	
      | 0.6399	
      | 0.6722	
      | 0.7035	
      | 0.7329	
      | 0.7619	
      | 0.7908	
      | 0.8182	
      | 0.8423	
      | 0.8591	
      | 0.8671	
      | 0.8694	
      | 0.87	
      | 0.8716	
      | 0.8748]
      Table=|
      | [-58.0321	
      | -41.3127	
      | -25.806	
      | -18.8199	
      | -18.1792	
      | -19.3912	
      | -20.4908	
      | -21.2523	
      | -21.637	
      | -21.5293	
      | -21.2147	
      | -21.1026	
      | -21.2255	
      | -21.0005	
      | -20.0862	
      | -18.9117	
      | -18.0033	
      | -17.2863	
      | -16.3901	
      | -15.3991	
      | -14.6918	
      | -14.2288	
      | -13.5974	
      | -12.7383	
      | -12.0772	
      | -11.8522	
      | -12.0927	
      | -12.3515	
      | -11.908	
      | -10.527	
      | -8.4461	
      | -6.1711	
      | -4.569	
      | -4.3374	
      | -4.9474	
      | -5.1203	
      | -4.1986	
      | -1.9655	
      | 1.4481	
      | 5.1672	
      | 8.1363	
      | 9.6899	
      | 9.8527	
      | 9.2903	
      | 8.9068	
      | 9.3854	
      | 10.0671	
      | 9.9786	
      | 9.566	
      | 9.4065	
      | 9.7211	
      | 10.9028	
      | 12.9299	
      | 14.8694	
      | 15.7043	
      | 15.818	
      | 15.5638	
      | 15.1851	
      | 15.3097	
      | 16.2461	
      | 17.5046	
      | 18.3783	
      | 18.4534	
      | 17.8871	
      | 17.4539	
      | 17.6379	
      | 18.1546	
      | 18.575	
      | 18.6821	
      | 18.5423	
      | 18.18	
      | 17.7569	
      | 18.1501	
      | 20.4906	
      | 25.6845	
      | 36.0276	
      | 55.1836	
      | 84.2363]
  Torque : Outport
  wires:
  Torque (in-lbs)/1 -> Torque/1
  Aileron Surface/1 -> Aileron Trim Position (in)/1
  Spring Delta (in)/1 -> Torque (in-lbs)/1
  Trim Position/1 -> Spring Delta (in)/2
  Aileron Trim Position (in)/1 -> Spring Delta (in)/1
